simulink model "vehicle_subsystems"  (R2015a)
settings: Solver=ode23t  StartTime=0.0  StopTime=300  RelTol=1e-3  AbsTol=1e-3
undefined symbols (not defined in the file): rider_mass, tire_dia, vehicle_mass
libraries: fl_lib x7, nesl_utility x5, sdl_lib x3
settings Model: Creator=sseshadr  LastModifiedBy=sseshadr
settings SimscapeCC: SimscapeLogType=all  SimscapeLogDataHistory=10000

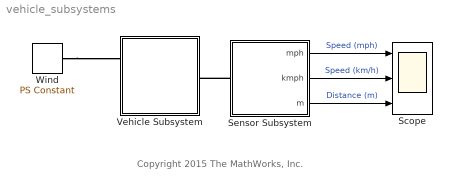
== system vehicle_subsystems ==
  note: Copyright 2015 The MathWorks, Inc.
  Scope : Scope  NumInputPorts=3
      settings: YMin=-5~-5~-5  YMax=5~5~5
  Sensor Subsystem : Subsystem
  Vehicle Subsystem : Subsystem
  Wind : fl_lib/Physical Signals/Sources/PS Constant  constant=1
  wires:
  Sensor Subsystem/1(mph) -> Scope/1  "Speed (mph)"
  Sensor Subsystem/2(kmph) -> Scope/2  "Speed (km/h)"
  Sensor Subsystem/3(m) -> Scope/3  "Distance (m)"
  connections:
  Sensor Subsystem/LConn1 -- Vehicle Subsystem/RConn1
  Wind/RConn1 -- Vehicle Subsystem/LConn1

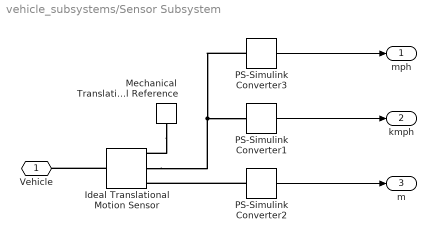
== system vehicle_subsystems/Sensor Subsystem ==
  Ideal Translational Motion Sensor : fl_lib/Mechanical/Mechanical Sensors/Ideal Translational Motion Sensor  offset=0 m
  Mechanical Translational Reference : fl_lib/Mechanical/Translational Elements/Mechanical Translational Reference
  PS-Simulink Converter1 : nesl_utility/PS-Simulink Converter  PhysicalDomain=network_engine_domain  SubClassName=ps_output  LeftPortType=input  RightPortType=output  PseudoPeriodic=off  Frequencies=[]  Unit=km/hr  AffineConversion=off
  PS-Simulink Converter2 : nesl_utility/PS-Simulink Converter  PhysicalDomain=network_engine_domain  SubClassName=ps_output  LeftPortType=input  RightPortType=output  PseudoPeriodic=off  Frequencies=[]  Unit=1  AffineConversion=off
  PS-Simulink Converter3 : nesl_utility/PS-Simulink Converter  PhysicalDomain=network_engine_domain  SubClassName=ps_output  LeftPortType=input  RightPortType=output  PseudoPeriodic=off  Frequencies=[]  Unit=mph  AffineConversion=off
  Vehicle : PMIOPort  Port=1  Side=Left
  mph : Outport
  kmph : Outport  Port=2
  m : Outport  Port=3
  wires:
  PS-Simulink Converter1/1 -> kmph/1
  PS-Simulink Converter2/1 -> m/1
  PS-Simulink Converter3/1 -> mph/1
  connections:
  Mechanical Translational Reference/LConn1 -- Ideal Translational Motion Sensor/RConn1
  PS-Simulink Converter2/LConn1 -- Ideal Translational Motion Sensor/RConn3
  Ideal Translational Motion Sensor/RConn2 -- PS-Simulink Converter3/LConn1 -- PS-Simulink Converter1/LConn1
  Ideal Translational Motion Sensor/LConn1 -- Vehicle/RConn1

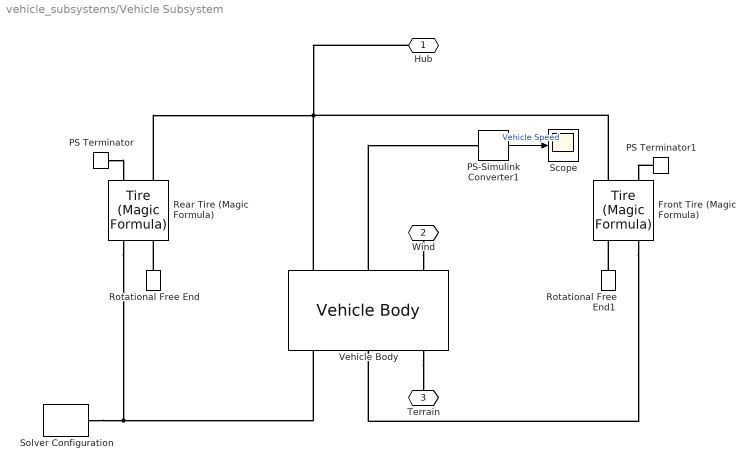
== system vehicle_subsystems/Vehicle Subsystem ==
  Front Tire (Magic Formula) : sdl_lib/Tires & Vehicles/Tire (Magic Formula)  parameterization=2  F_z1=3e+3 N  F_x1=3.5e+3 N  kappa1=10  B_m=tire_b  C_m=tire_c  D_m=tire_d  E_m=tire_e  fz0=4e+3 N  p_Cx=1.685  p_Dx=[ 1.21 -0.037 ]  p_Ex=[ 0.344 0.095 -0.02 0 ]  p_Kx=[ 21.51 -0.163 0.245 ]  p_Hx=[ -0.002 0.002 ]  p_Vx=[ 0 0 ]  v_tr_thr=0.1 m/s  r_e=tire_dia/2 in  model_compliance=0  stiffness=1e+6 N/m  damping=1000 N/(m/s)  model_inertia=1  inertia=tire_inertia kg*m^2  initial_velocity=0 rad/s  model_resistance=1  resistance_model=1  coeff=roll_resist  p_tire=250e3 Pa  alpha=-0.003  beta=0.97  coeff_a=84e-4  coeff_b=6.2e-4 s/m  coeff_c=1.6e-4 s^2/m^2  v_thr=1e-3 m/s
  PS Terminator : fl_lib/Physical Signals/Sinks/PS Terminator
  PS Terminator1 : fl_lib/Physical Signals/Sinks/PS Terminator
  PS-Simulink Converter1 : nesl_utility/PS-Simulink Converter  PhysicalDomain=network_engine_domain  SubClassName=ps_output  LeftPortType=input  RightPortType=output  PseudoPeriodic=off  Frequencies=[]  Unit=1  AffineConversion=off
  Rear Tire (Magic Formula) : sdl_lib/Tires & Vehicles/Tire (Magic Formula)  parameterization=2  F_z1=3e+3 N  F_x1=3.5e+3 N  kappa1=10  B_m=tire_b  C_m=tire_c  D_m=tire_d  E_m=tire_e  fz0=4e+3 N  p_Cx=1.685  p_Dx=[ 1.21 -0.037 ]  p_Ex=[ 0.344 0.095 -0.02 0 ]  p_Kx=[ 21.51 -0.163 0.245 ]  p_Hx=[ -0.002 0.002 ]  p_Vx=[ 0 0 ]  v_tr_thr=0.1 m/s  r_e=tire_dia/2 in  model_compliance=0  stiffness=1e+6 N/m  damping=1000 N/(m/s)  model_inertia=1  inertia=tire_inertia kg*m^2  initial_velocity=0 rad/s  model_resistance=1  resistance_model=1  coeff=roll_resist  p_tire=250e3 Pa  alpha=-0.003  beta=0.97  coeff_a=84e-4  coeff_b=6.2e-4 s/m  coeff_c=1.6e-4 s^2/m^2  v_thr=1e-3 m/s
  Rotational Free End : fl_lib/Mechanical/Rotational Elements/Rotational Free End  w_specify=off  w_priority=High  w=0 rad/s
  Rotational Free End1 : fl_lib/Mechanical/Rotational Elements/Rotational Free End  w_specify=off  w_priority=High  w=0 rad/s
  Scope : Scope
  Solver Configuration : nesl_utility/Solver Configuration  PhysicalDomain=network_engine_domain  SubClassName=solver  LeftPortType=input  RightPortType=generic  Accelerate=off  Tones=[]  Harmonics=[]  SimulateNoise=off  Profile=off  UseLocalSampling=off  EnableSwitchedLinearOptims=on  FrequencyDomain=off  UseCCode=off  RelTol=0.001  AbsTol=1e-06  MinStep=1e-09  ToWorkspace=off  RevertToSquareIcSolve=off  NumHomotopyIterations=100  DoDC=off  ResidualTolerance=1e-09  UseLocalSolver=off  LocalSolverChoice=NE_BACKWARD_EULER_ADVANCER  LocalSolverSampleTime=0.001  DoFixedCost=off  MaxNonlinIter=3  MaxModeIter=2  LinearAlgebra=Sparse  DelaysMemoryBudget=1024  AutomaticFiltering=on  FilteringTimeConstant=0.001
  Vehicle Body : sdl_lib/Tires & Vehicles/Vehicle Body  mass=rider_mass + vehicle_mass kg  n_w=1  x_f=front_axle mm  x_r=rear_axle mm  y_c=CG_height mm  area=front_area m^2  Cd=drag_coeff  v0=0 m/s  g=9.81 m/s^2  rho=1.18 kg/m^3
  Hub : PMIOPort  Port=1  Side=Right
  Wind : PMIOPort  Port=2  Side=Left
  Terrain : PMIOPort  Port=3  Side=Left
  wires:
  PS-Simulink Converter1/1 -> Scope/1  "Vehicle Speed"
  connections:
  Rear Tire (Magic Formula)/LConn1 -- Solver Configuration/RConn1 -- Vehicle Body/RConn1
  Front Tire (Magic Formula)/RConn2 -- Hub/RConn1 -- Rear Tire (Magic Formula)/RConn2 -- Vehicle Body/LConn1
  PS Terminator/LConn1 -- Rear Tire (Magic Formula)/RConn1
  Rotational Free End1/LConn1 -- Front Tire (Magic Formula)/LConn2
  Front Tire (Magic Formula)/LConn1 -- Vehicle Body/RConn2
  Rotational Free End/LConn1 -- Rear Tire (Magic Formula)/LConn2
  Vehicle Body/RConn3 -- Terrain/RConn1
  PS Terminator1/LConn1 -- Front Tire (Magic Formula)/RConn1
  Vehicle Body/LConn2 -- PS-Simulink Converter1/LConn1
  Wind/RConn1 -- Vehicle Body/LConn3
